simulink model "sec2_c"  (R2018b)
settings: Solver=VariableStepAuto  StartTime=0.0  StopTime=0.8  MaxStep=0.001  RelTol=1e-3
settings Model: Creator=buddyugwumba1  LastModifiedBy=buddyugwumba1

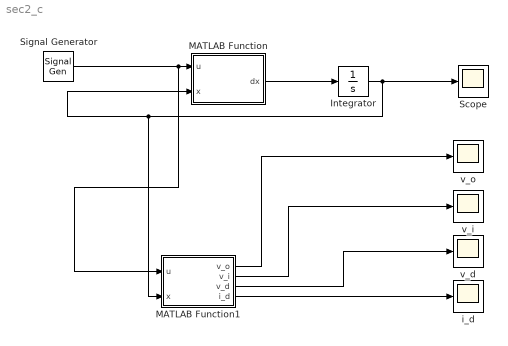
== system sec2_c ==
  Integrator : Integrator
  MATLAB Function : MATLAB Function  TreatAsAtomicUnit=on
  MATLAB Function1 : MATLAB Function  TreatAsAtomicUnit=on
  Scope : Scope
  Signal Generator : SignalGenerator  Amplitude=120  Frequency=2*pi*60  Units=rad/sec
  i_d : Scope
  v_d : Scope
  v_i : Scope
  v_o : Scope
  wires:
  Signal Generator/1 -> MATLAB Function1/1(u), MATLAB Function/1(u)
  MATLAB Function/1(dx) -> Integrator/1
  Integrator/1 -> Scope/1, MATLAB Function1/2(x), MATLAB Function/2(x)
  MATLAB Function1/4(i_d) -> i_d/1
  MATLAB Function1/3(v_d) -> v_d/1
  MATLAB Function1/2(v_i) -> v_i/1
  MATLAB Function1/1(v_o) -> v_o/1

== matlab function sec2_c/MATLAB Function1 ==
  data: u input; v_o output; x input; v_i output; v_d output; i_d output
function [v_o,v_i,v_d,i_d] = fcn(u, x)

R = 1000;
N = 10;
v_o = x(4)*R;
v_i = x(1);
v_d = (u/N - x(1));
i_d = diode(v_d);
end

== matlab function sec2_c/MATLAB Function ==
  data: u input; dx output; x input
function dx = fcn(u, x)
%DX Summary of this function goes here
%   Detailed explanation goes here
R = 1000;
C = 100e-6;
L = 0.7793;
N = 10;
v_d = (u/N - x(1));
dx = zeros(4,1);
dx(1) = -1/C*x(2) + 1/C*diode(v_d);
dx(2) = 1/L*x(1) - 1/L*x(3);
dx(3) = 1/C*x(2) - 1/C*x(4);
dx(4) = 1/L*x(3) - R/L*x(4);
end
